simulink model "Modele_Lineaire_Asservi"  (R2024a)
settings: Solver=VariableStepAuto  StartTime=0.0  StopTime=10  RelTol=1e-3
values from neighbouring files (symbols this model uses):
  den_bille_simu = [7*L 0]    [Initialisation.m]
  den_mot_simu = [R_m*J_eq  (R_m*B_eq+n_g*n_m*k_m*k_t*K_g.^2)]    [Initialisation.m]
  K_int = real((((-1)*den_mot(1)*(Inter^2)) + ((-1)*den_mot(2)*(Inter^1))) / (num_mot(1)))    [Initialisation.m]
  num_bille_simu = [5*g*r_arm]    [Initialisation.m]
  num_mot_simu = [K_g*n_m*n_g*k_t]    [Initialisation.m]
  Test_Position = 0.06    [Initialisation.m]
  X_den = TF_PD_Bode_Den    [Initialisation.m]
  X_num = TF_PD_Bode_Num    [Initialisation.m]
settings Model: Creator=francoisdesautels  LastModifiedBy=francoisdesautels

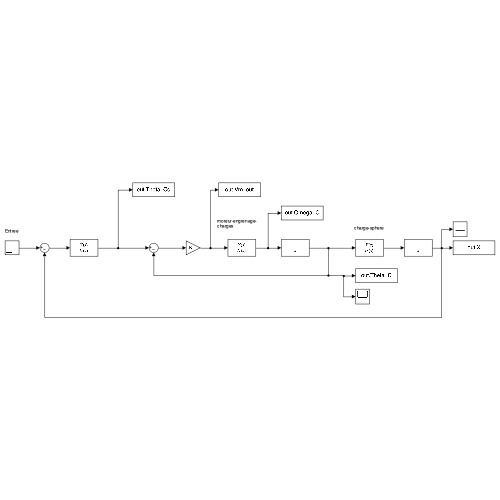
[thumbnail: Simulink's stored preview of the top-level diagram]
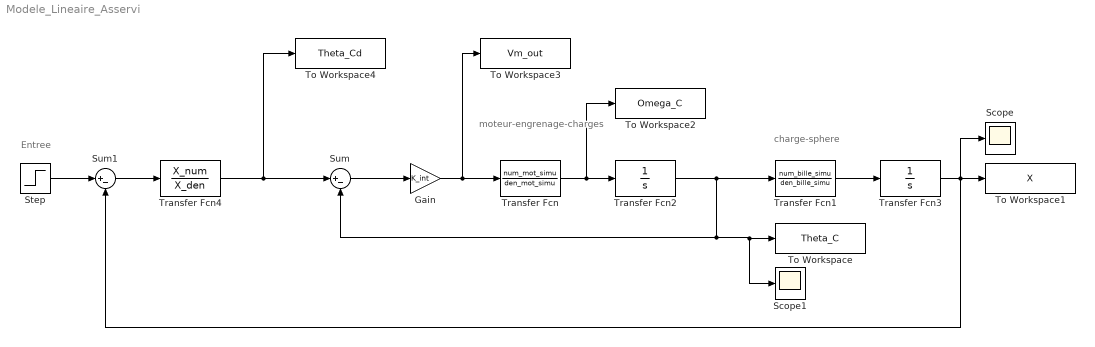
== system Modele_Lineaire_Asservi ==
  note: charge-sphere
  note: moteur-engrenage-charges
  note: Entree
  Gain : Gain  Gain=K_int
  Scope : Scope
  Scope1 : Scope
  Step : Step  After=Test_Position  SampleTime=0
  Sum : Sum  Inputs=|+-
  Sum1 : Sum  Inputs=|+-
  To Workspace : ToWorkspace  VariableName=Theta_C  SaveFormat=Timeseries  SampleTime=-1
      settings: Save2DSignal=2-D array (concatenate along first dimension)
  To Workspace1 : ToWorkspace  VariableName=X  SaveFormat=Timeseries  SampleTime=-1
  To Workspace2 : ToWorkspace  VariableName=Omega_C  SaveFormat=Timeseries  SampleTime=-1
  To Workspace3 : ToWorkspace  VariableName=Vm_out  SaveFormat=Timeseries  SampleTime=-1
      settings: Save2DSignal=2-D array (concatenate along first dimension)
  To Workspace4 : ToWorkspace  VariableName=Theta_Cd  SaveFormat=Timeseries  SampleTime=-1
      settings: Save2DSignal=2-D array (concatenate along first dimension)
  Transfer Fcn : TransferFcn  Numerator=num_mot_simu  Denominator=den_mot_simu
  Transfer Fcn1 : TransferFcn  Numerator=num_bille_simu  Denominator=den_bille_simu
  Transfer Fcn2 : TransferFcn  Denominator=[1 0]
  Transfer Fcn3 : TransferFcn  Denominator=[1 0]
  Transfer Fcn4 : TransferFcn  Numerator=X_num  Denominator=X_den
  wires:
  Transfer Fcn/1 -> To Workspace2/1, Transfer Fcn2/1
  Transfer Fcn1/1 -> Transfer Fcn3/1
  Transfer Fcn2/1 -> Scope1/1, To Workspace/1, Sum/2, Transfer Fcn1/1
  Transfer Fcn3/1 -> Sum1/2, To Workspace1/1, Scope/1
  Sum/1 -> Gain/1
  Gain/1 -> To Workspace3/1, Transfer Fcn/1
  Transfer Fcn4/1 -> To Workspace4/1, Sum/1
  Step/1 -> Sum1/1
  Sum1/1 -> Transfer Fcn4/1
